simulink library "libo_robotics"  (R2015b)
settings: Solver=ode1  StartTime=0.0  StopTime=Inf  FixedStep=0.001  RelTol=1e-3
PostLoadFcn:
  | , if any(exist('dsrtsu_mdlpostloadfcn', 'file') == [2, 3, 6]), try dsrtsu_mdlpostloadfcn('Execute', bdroot); catch fprintf('Error in PostLoadFcn (dsrtsu_mdlpostloadfcn) for model "%s":\n %s\n', bdroot, lasterr); end, end,
libraries: libo_robotics x2
settings Model: DSRTSU_INTERNAL_RTI_VER=440  DSRTSU_INTERNAL_RTI_TYPE=rti1007  DSRTSU_INTERNAL_RTIFPGA=30  Creator=Mahl  LastModifiedBy=Mayer
settings DataIOCC: SaveFormat=Array  SignalLoggingSaveFormat=ModelDataLogs
settings OptimizationCC: BlockReduction=off  OptimizeBlockIOStorage=off  BufferReuse=off  GlobalBufferReuse=off  ExpressionFolding=off  ExpressionDepthLimit=2147483647  LocalBlockOutputs=off
settings DebuggingCC: UnderspecifiedInitializationDetection=Classic  MergeDetectMultiDrivingBlocksExec=none  SolverPrmCheckMsg=warning  FcnCallInpInsideContextMsg=UseLocalSettings  StateNameClashWarn=warning
settings HardwareCC: ProdBitPerPointer=32  ProdLargestAtomicFloat=None  ProdEndianess=BigEndian  ProdWordSize=32  ProdHWDeviceType=Generic->Custom  TargetIntDivRoundTo=Zero  TargetEndianess=BigEndian  TargetHWDeviceType=Generic->Custom
settings RTWCC: SystemTargetFile=rti1103.tlc  MakeCommand=make_rti  TemplateMakefile=rti1103.tmf  Description=dSPACE DS1103 Hardware Platform
settings STFCustomTargetCC: ParMdlRefBuildCompliant=on  ConcurrentExecutionCompliant=off  MatFileLogging=on  SystemTargetFile=rti1103.tlc
settings GRTTargetCC: CompOptLevelCompliant=off  ConcurrentExecutionCompliant=off  GeneratePreprocessorConditionals=Disable all  CombineOutputUpdateFcns=off  GRTInterface=on  UseToolchainInfoCompliant=off  ExtModeMexFile=noextcomm
settings ConfigComp: CovModelRefEnable=Off

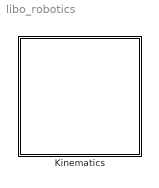
== system libo_robotics ==
  Kinematics : Subsystem

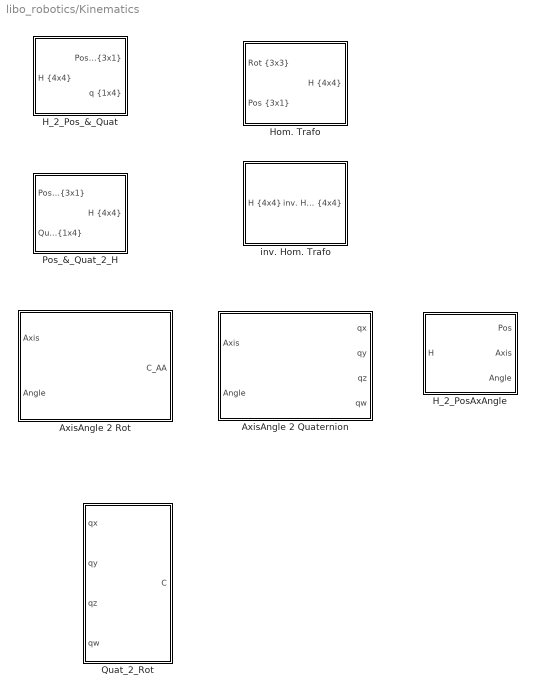
== system libo_robotics/Kinematics ==
  AxisAngle 2 Quaternion : MATLAB Function  TreatAsAtomicUnit=on
  AxisAngle 2 Rot : MATLAB Function  TreatAsAtomicUnit=on
  H_2_PosAxAngle : MATLAB Function  TreatAsAtomicUnit=on
  H_2_Pos_&_Quat : Subsystem
  Hom. Trafo : Subsystem
  Pos_&_Quat_2_H : Subsystem
  Quat_2_Rot : Subsystem
  inv. Hom. Trafo : Subsystem

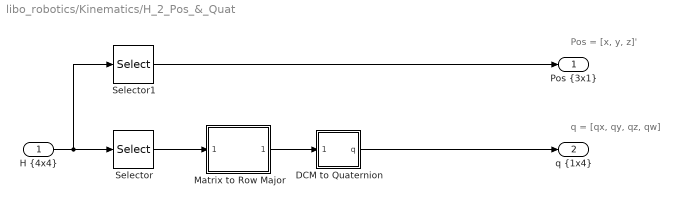
== system libo_robotics/Kinematics/H_2_Pos_&_Quat ==
  note: Pos = [x, y, z]'
  note: q = [qx, qy, qz, qw]
  "H {4x4}" : Inport
  DCM to Quaternion : Subsystem  mask(DCM to Quaternion){}
      mask help:
      | Converts a direction cosine matrix (DCM) to a quaternion that would perform the equivalent vector transformation, i.e., q*vq = Rv, where R is the DCM, v is a vector, and q is the quaternion.
      |
      | Note that for purposes of quaternion-vector multiplication, a vector is treated as a quaterion with a scalar element of zero.
  Matrix to Row Major : Subsystem  mask(Matrix to Row Major){}
      mask help: Converts a matrix to row major vector form.
      mask Display: fprintf('Matrix to\nRow Major');
  Selector : Selector  NumberOfDimensions=2  InputPortWidth=3  IndexOptions=Index vector (dialog),Index vector (dialog)  Indices=[1 2 3],[1 2 3]  OutputSizes=1,1
  Selector1 : Selector  NumberOfDimensions=2  InputPortWidth=3  IndexOptions=Index vector (dialog),Index vector (dialog)  Indices=[1 2 3],4  OutputSizes=1,1
  "Pos {3x1}" : Outport
  "q {1x4}" : Outport  Port=2
  wires:
  Matrix to Row Major/1(vector) -> DCM to Quaternion/1(DCM)
  DCM to Quaternion/1(q) -> "q {1x4}"/1
  Selector/1 -> Matrix to Row Major/1(matrix)
  "H {4x4}"/1 -> Selector/1, Selector1/1
  Selector1/1 -> "Pos {3x1}"/1

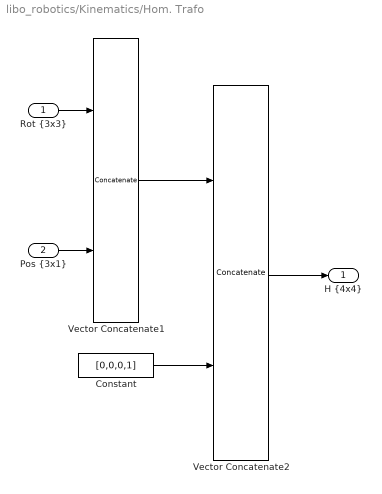
== system libo_robotics/Kinematics/Hom. Trafo ==
  "Rot {3x3}" : Inport
  "Pos {3x1}" : Inport  Port=2
  Constant : Constant  Value=[0,0,0,1]  VectorParams1D=off
  Vector Concatenate1 : Concatenate  Mode=Multidimensional array  ConcatenateDimension=2
  Vector Concatenate2 : Concatenate  Mode=Multidimensional array
  "H {4x4}" : Outport
  wires:
  Vector Concatenate2/1 -> "H {4x4}"/1
  Constant/1 -> Vector Concatenate2/2
  Vector Concatenate1/1 -> Vector Concatenate2/1
  "Rot {3x3}"/1 -> Vector Concatenate1/1
  "Pos {3x1}"/1 -> Vector Concatenate1/2

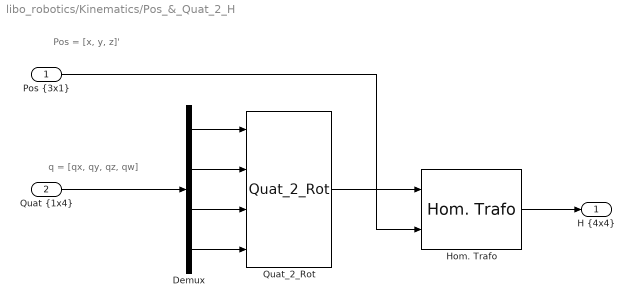
== system libo_robotics/Kinematics/Pos_&_Quat_2_H ==
  note: q = [qx, qy, qz, qw]
  note: Pos = [x, y, z]'
  "Pos {3x1}" : Inport
  "Quat {1x4}" : Inport  Port=2
  Demux : Demux
  Hom. Trafo : libo_robotics/Kinematics/Hom. Trafo
  Quat_2_Rot : libo_robotics/Kinematics/Quat_2_Rot
  "H {4x4}" : Outport
  wires:
  "Quat {1x4}"/1 -> Demux/1
  Quat_2_Rot/1 -> Hom. Trafo/1
  "Pos {3x1}"/1 -> Hom. Trafo/2
  Hom. Trafo/1 -> "H {4x4}"/1
  Demux/1 -> Quat_2_Rot/1
  Demux/2 -> Quat_2_Rot/2
  Demux/3 -> Quat_2_Rot/3
  Demux/4 -> Quat_2_Rot/4

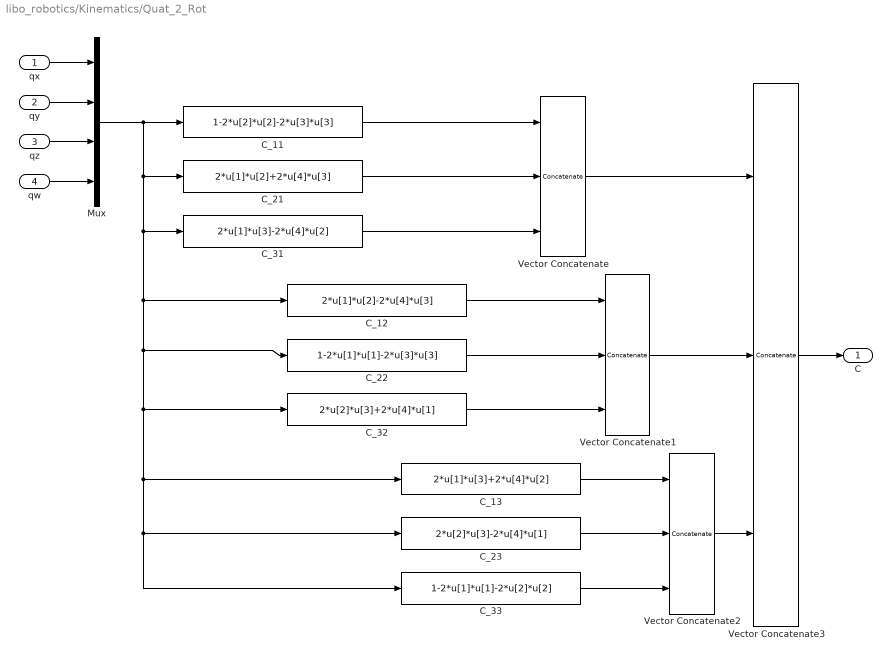
== system libo_robotics/Kinematics/Quat_2_Rot ==
  qx : Inport
  qy : Inport  Port=2
  qz : Inport  Port=3
  qw : Inport  Port=4
  C_11 : Fcn  Expr=1-2*u[2]*u[2]-2*u[3]*u[3]
  C_12 : Fcn  Expr=2*u[1]*u[2]-2*u[4]*u[3]
  C_13 : Fcn  Expr=2*u[1]*u[3]+2*u[4]*u[2]
  C_21 : Fcn  Expr=2*u[1]*u[2]+2*u[4]*u[3]
  C_22 : Fcn  Expr=1-2*u[1]*u[1]-2*u[3]*u[3]
  C_23 : Fcn  Expr=2*u[2]*u[3]-2*u[4]*u[1]
  C_31 : Fcn  Expr=2*u[1]*u[3]-2*u[4]*u[2]
  C_32 : Fcn  Expr=2*u[2]*u[3]+2*u[4]*u[1]
  C_33 : Fcn  Expr=1-2*u[1]*u[1]-2*u[2]*u[2]
  Mux : Mux
  Vector Concatenate : Concatenate  NumInputs=3  Mode=Multidimensional array
  Vector Concatenate1 : Concatenate  NumInputs=3  Mode=Multidimensional array
  Vector Concatenate2 : Concatenate  NumInputs=3  Mode=Multidimensional array
  Vector Concatenate3 : Concatenate  NumInputs=3  Mode=Multidimensional array  ConcatenateDimension=2
  C : Outport
  wires:
  qx/1 -> Mux/1
  qy/1 -> Mux/2
  qz/1 -> Mux/3
  qw/1 -> Mux/4
  Mux/1 -> C_33/1, C_23/1, C_13/1, C_32/1, C_22/1, C_12/1, C_31/1, C_21/1, C_11/1
  C_11/1 -> Vector Concatenate/1
  C_21/1 -> Vector Concatenate/2
  C_31/1 -> Vector Concatenate/3
  C_12/1 -> Vector Concatenate1/1
  C_22/1 -> Vector Concatenate1/2
  C_32/1 -> Vector Concatenate1/3
  C_13/1 -> Vector Concatenate2/1
  C_23/1 -> Vector Concatenate2/2
  C_33/1 -> Vector Concatenate2/3
  Vector Concatenate/1 -> Vector Concatenate3/1
  Vector Concatenate1/1 -> Vector Concatenate3/2
  Vector Concatenate2/1 -> Vector Concatenate3/3
  Vector Concatenate3/1 -> C/1

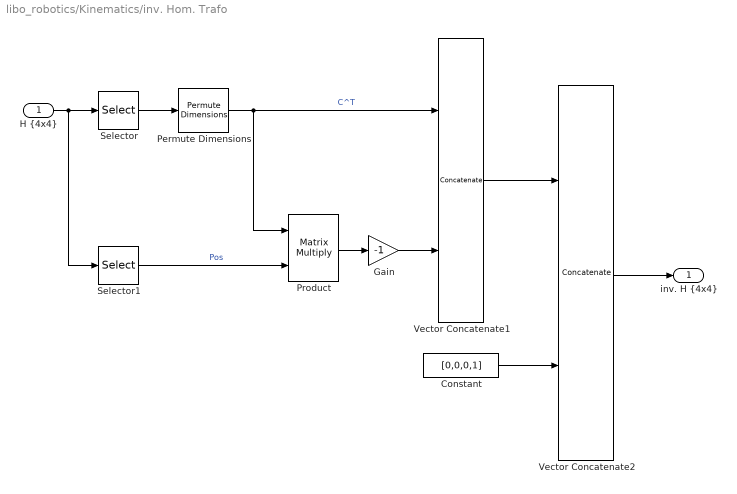
== system libo_robotics/Kinematics/inv. Hom. Trafo ==
  "H {4x4}" : Inport
  Constant : Constant  Value=[0,0,0,1]  VectorParams1D=off
  Gain : Gain  Gain=-1
  Permute Dimensions : PermuteDimensions
  Product : Product  Multiplication=Matrix(*)  RndMeth=Zero
  Selector : Selector  NumberOfDimensions=2  InputPortWidth=3  IndexOptions=Index vector (dialog),Index vector (dialog)  Indices=[1 2 3],[1 2 3]  OutputSizes=1,1
  Selector1 : Selector  NumberOfDimensions=2  InputPortWidth=3  IndexOptions=Index vector (dialog),Index vector (dialog)  Indices=[1 2 3],[4]  OutputSizes=1,1
  Vector Concatenate1 : Concatenate  Mode=Multidimensional array  ConcatenateDimension=2
  Vector Concatenate2 : Concatenate  Mode=Multidimensional array
  "inv. H {4x4}" : Outport
  wires:
  Vector Concatenate1/1 -> Vector Concatenate2/1
  Constant/1 -> Vector Concatenate2/2
  Vector Concatenate2/1 -> "inv. H {4x4}"/1
  "H {4x4}"/1 -> Selector/1, Selector1/1
  Selector/1 -> Permute Dimensions/1
  Permute Dimensions/1 -> Vector Concatenate1/1, Product/1  "C^T"
  Product/1 -> Gain/1
  Selector1/1 -> Product/2  "Pos"
  Gain/1 -> Vector Concatenate1/2

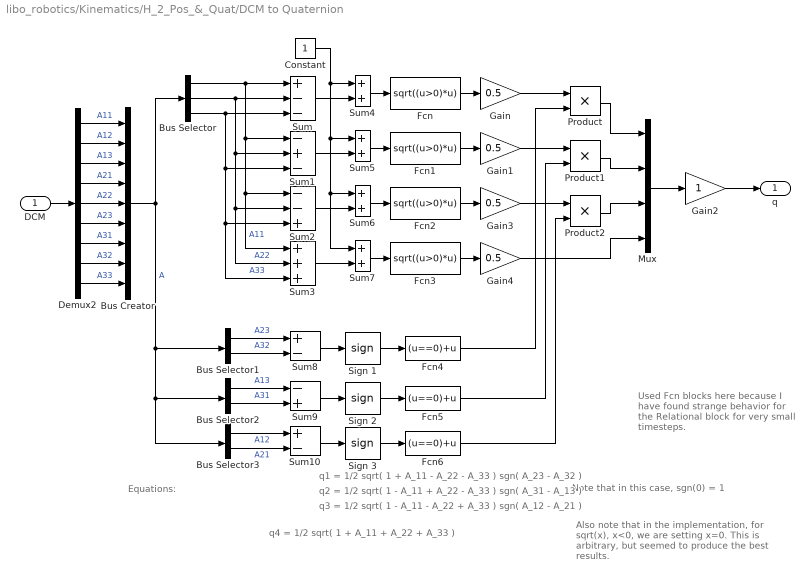
== system libo_robotics/Kinematics/H_2_Pos_&_Quat/DCM to Quaternion ==
  note: Also note that in the implementation,
      | for sqrt(x), x<0, we are setting x=0.
      | This is arbitrary, but seemed to produce
      | the best results.
  note: Note that in this case, sgn(0) = 1
  note: Equations:
  note: q4 = 1/2 sqrt( 1 + A_11 + A_22 + A_33 )
  note: q3 = 1/2 sqrt( 1 - A_11 - A_22 + A_33 ) sgn( A_12 - A_21 )
  note: q2 = 1/2 sqrt( 1 - A_11 + A_22 - A_33 ) sgn( A_31 - A_13 )
  note: q1 = 1/2 sqrt( 1 + A_11 - A_22 - A_33 ) sgn( A_23 - A_32 )
  note: Used Fcn blocks here because
      | I have found strange behavior
      | for the Relational block for
      | very small timesteps.
  DCM : Inport  PortDimensions=9
  Bus Creator : BusCreator  Inputs=9
  Bus Selector : BusSelector  OutputSignals=A11,A22,A33
  Bus Selector1 : BusSelector  OutputSignals=A23,A32
  Bus Selector2 : BusSelector  OutputSignals=A13,A31
  Bus Selector3 : BusSelector  OutputSignals=A12,A21
  Constant : Constant
  Demux2 : Demux  Outputs=9
  Fcn{,1..3} (4 alike) : Fcn  Expr=sqrt((u>0)*u)
  Fcn4 : Fcn  Expr=(u==0)+u
  Fcn5 : Fcn  Expr=(u==0)+u
  Fcn6 : Fcn  Expr=(u==0)+u
  Gain{,1,3..4} (4 alike) : Gain  Gain=0.5  SaturateOnIntegerOverflow=on  OutDataTypeStr=Inherit: Same as input  ParamDataTypeStr=Inherit: Same as input
  Gain2 : Gain  SaturateOnIntegerOverflow=on  OutDataTypeStr=Inherit: Same as input  ParamDataTypeStr=Inherit: Same as input
  Mux : Mux
  Product : Product  SaturateOnIntegerOverflow=on  RndMeth=Zero  InputSameDT=on  OutDataTypeStr=Inherit: Same as first input
  Product1 : Product  SaturateOnIntegerOverflow=on  RndMeth=Zero  InputSameDT=on  OutDataTypeStr=Inherit: Same as first input
  Product2 : Product  SaturateOnIntegerOverflow=on  RndMeth=Zero  InputSameDT=on  OutDataTypeStr=Inherit: Same as first input
  Sign 1 : Signum
  Sign 2 : Signum
  Sign 3 : Signum
  Sum : Sum  Inputs=+--  SaturateOnIntegerOverflow=on  InputSameDT=on  OutDataTypeStr=Inherit: Same as first input
  Sum1 : Sum  Inputs=-+-  SaturateOnIntegerOverflow=on  InputSameDT=on  OutDataTypeStr=Inherit: Same as first input
  Sum10 : Sum  Inputs=+-  SaturateOnIntegerOverflow=on  InputSameDT=on  OutDataTypeStr=Inherit: Same as first input
  Sum2 : Sum  Inputs=--+  SaturateOnIntegerOverflow=on  InputSameDT=on  OutDataTypeStr=Inherit: Same as first input
  Sum3 : Sum  Inputs=+++  SaturateOnIntegerOverflow=on  InputSameDT=on  OutDataTypeStr=Inherit: Same as first input
  Sum{4..7} (4 alike) : Sum  SaturateOnIntegerOverflow=on  InputSameDT=on  OutDataTypeStr=Inherit: Same as first input
  Sum8 : Sum  Inputs=+-  SaturateOnIntegerOverflow=on  InputSameDT=on  OutDataTypeStr=Inherit: Same as first input
  Sum9 : Sum  Inputs=-+  SaturateOnIntegerOverflow=on  InputSameDT=on  OutDataTypeStr=Inherit: Same as first input
  q : Outport  InitialOutput=[0 0 0 1]
  wires:
  Mux/1 -> Gain2/1
  Gain4/1 -> Mux/4
  Product2/1 -> Mux/3
  Product1/1 -> Mux/2
  Product/1 -> Mux/1
  Bus Creator/1 -> Bus Selector3/1, Bus Selector2/1, Bus Selector1/1, Bus Selector/1  "A"
  DCM/1 -> Demux2/1
  Demux2/9 -> Bus Creator/9  "A33"
  Demux2/8 -> Bus Creator/8  "A32"
  Demux2/7 -> Bus Creator/7  "A31"
  Demux2/6 -> Bus Creator/6  "A23"
  Demux2/5 -> Bus Creator/5  "A22"
  Demux2/4 -> Bus Creator/4  "A21"
  Demux2/3 -> Bus Creator/3  "A13"
  Demux2/2 -> Bus Creator/2  "A12"
  Demux2/1 -> Bus Creator/1  "A11"
  Bus Selector3/1 -> Sum10/1  "A12"
  Bus Selector3/2 -> Sum10/2  "A21"
  Bus Selector2/2 -> Sum9/2  "A31"
  Bus Selector2/1 -> Sum9/1  "A13"
  Bus Selector/3 -> Sum2/3, Sum3/3, Sum1/3, Sum/3  "A33"
  Bus Selector/1 -> Sum3/1, Sum2/1, Sum1/1, Sum/1  "A11"
  Bus Selector/2 -> Sum2/2, Sum3/2, Sum1/2, Sum/2  "A22"
  Bus Selector1/2 -> Sum8/2  "A32"
  Bus Selector1/1 -> Sum8/1  "A23"
  Sign 3/1 -> Fcn6/1
  Fcn6/1 -> Product2/2
  Sum10/1 -> Sign 3/1
  Sign 2/1 -> Fcn5/1
  Fcn5/1 -> Product1/2
  Sum9/1 -> Sign 2/1
  Sign 1/1 -> Fcn4/1
  Fcn4/1 -> Product/2
  Sum8/1 -> Sign 1/1
  Fcn2/1 -> Gain3/1
  Fcn3/1 -> Gain4/1
  Fcn1/1 -> Gain1/1
  Fcn/1 -> Gain/1
  Sum7/1 -> Fcn3/1
  Sum6/1 -> Fcn2/1
  Sum5/1 -> Fcn1/1
  Gain3/1 -> Product2/1
  Gain1/1 -> Product1/1
  Gain/1 -> Product/1
  Sum2/1 -> Sum6/2
  Sum3/1 -> Sum7/2
  Sum4/1 -> Fcn/1
  Constant/1 -> Sum7/1, Sum6/1, Sum5/1, Sum4/1
  Sum1/1 -> Sum5/2
  Sum/1 -> Sum4/2
  Gain2/1 -> q/1

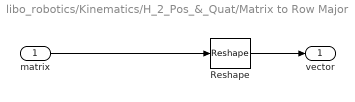
== system libo_robotics/Kinematics/H_2_Pos_&_Quat/Matrix to Row Major ==
  matrix : Inport
  Reshape : Reshape  OutputDimensions=[3, 3]
      settings: AttributesFormatString=Output: %<OutputDimensionality>
  vector : Outport
  wires:
  Reshape/1 -> vector/1
  matrix/1 -> Reshape/1

== matlab function libo_robotics/Kinematics/AxisAngle 2 Rot ==
  data: Axis input; C_AA output; Angle input
function C_AA = AxisAngle_2_Rot(Axis, Angle)

%XXXXXXXXXXXXXXXXXXXXXXXXXXXXXXXXXXXXXXXXXXXXXXXXXXXXXXXXXXXXXXXXXXXXXXXXXX
% Funktion zur Berechnung der Rotationsmatrix C für eine Drehung um die
% Achse Axis mit dem Winkel Angle
%
% Input:
%   Axis    3x1     [-]     Drehachse
%   Angle   1x1     [rad]   Drehwinkel
%
% Output:
%   C_AA    3x3     [-]     Rotationsmatrix
%XXXXXXXXXXXXXXXXXXXXXXXXXXXXXXXXXXXXXXXXXXXXXXXXXXXXXXXXXXXXXXXXXXXXXXXXXX

c = cos(Angle);
s = sin(Angle);

n = Axis./norm(Axis,2);

C_AA = [c+(n(1))^2*(1-c),           n(1)*n(2)*(1-c)-n(3)*s,     n(1)*n(3)*(1-c)+n(2)*s;
        n(1)*n(2)*(1-c)+n(3)*s,     c+(n(2))^2*(1-c),           n(2)*n(3)*(1-c)-n(1)*s;
        n(1)*n(3)*(1-c)-n(2)*s,     n(2)*n(3)*(1-c)+n(1)*s,     c+(n(3))^2*(1-c)];

== matlab function libo_robotics/Kinematics/H_2_PosAxAngle ==
  data: H input size=[4,4]; Pos output size=[3,1]; Axis output size=[3,1]; Angle output size=[1,1]
function [Pos, Axis, Angle] = fcn(H)
% Input:    
% - Homogene Transformationsmatrix H
% Output:
% - Position Pos
% - Drehachse Axis
% - Drehwinkel Angle

Pos     = H(1:3, 4);
Axis    = zeros(3,1);
Angle   = acos(min([1,max([-1,(H(1,1)+H(2,2)+H(3,3)-1)/2]),1]));

if abs(sin(Angle)) < 1e-6
    if abs(1-cos(Angle)) < 1e-6
        Axis = [1;0;0];
    else
        abs_x = sqrt((H(1,1)+1)/2);
        abs_y = sqrt((H(2,2)+1)/2);
        abs_z = sqrt((H(3,3)+1)/2);

        Axis = [abs_x;...
                abs_y * sign(H(1,2));...
                abs_z * sign(H(1,3))];
    end
else
    Axis = 1/(2*sin(Angle))*[H(3,2)-H(2,3);...
                             H(1,3)-H(3,1);...
                             H(2,1)-H(1,2)];
end

== matlab function libo_robotics/Kinematics/AxisAngle 2 Quaternion ==
  data: Axis input; qx output; Angle input; qy output; qz output; qw output
function [qx, qy, qz, qw] = AxisAngle_2_Quaternion(Axis, Angle)
%#eml

n = Axis./norm(Axis,2);

qx = n(1)*sin(Angle/2);
qy = n(2)*sin(Angle/2);
qz = n(3)*sin(Angle/2);
qw = cos(Angle/2);
